simulink model "ball_and_plate_za_nn_2"  (R2018b)
settings: Solver=ode45  StartTime=0.0  StopTime=t_sim  RelTol=1e-3  EnableMultiTasking=on
values from neighbouring files (symbols this model uses):
  A_x = 0.05    [parametri.mat]    (also in proba_nn_simulink.m = 0.1; simulate_NOE_NARX_performance.mat = 0.1; simuliraj_kruznicu.m = radijus; test_nn_.m = 0.1)
  a_x = 0.388    [parametri.mat]    (also in simulate_NOE_NARX_performance.mat)
  A_y = 0.05    [parametri.mat]    (also in proba_nn_simulink.m = 0.1; simulate_NOE_NARX_performance.mat = 0.1; simuliraj_kruznicu.m = radijus; test_nn_.m = 0.1)
  a_y = 0.473    [parametri.mat]    (also in simulate_NOE_NARX_performance.mat)
  Ak_x = 0.1    [parametri.mat]    (also in simulate_NOE_NARX_performance.mat; simuliraj_kvadrat.m = stranica)
  Ak_y = 0.1    [parametri.mat]    (also in simulate_NOE_NARX_performance.mat; simuliraj_kvadrat.m = stranica)
  d = 2    [parametri.mat]    (also in simulate_NOE_NARX_performance.mat)
  Fc = 9.9675e-08    [parametri.mat]    (also in simulate_NOE_NARX_performance.mat)
  freq_x = 0.628318530718    [parametri.mat]    (also in simulate_NOE_NARX_performance.mat)
  freq_y = 0.628318530718    [parametri.mat]    (also in simulate_NOE_NARX_performance.mat)
  Fs = 1.9935e-07    [parametri.mat]    (also in simulate_NOE_NARX_performance.mat)
  g = 9.81    [parametri.mat]    (also in simulate_NOE_NARX_performance.mat)
  Jl = 7.48815837481e-05    [parametri.mat]    (also in simulate_NOE_NARX_performance.mat)
  konstanta = 0.1    [parametri.mat]    (also in simulate_NOE_NARX_performance.mat; simuliraj_kvadrat.m = 0.03)
  l = 0.1    [parametri.mat]    (also in simulate_NOE_NARX_performance.mat)
  ml = 0.0786597330257    [parametri.mat]    (also in simulate_NOE_NARX_performance.mat)
  odabir = 3    [proba_nn_simulink.m]    (also in simulate_NOE_NARX_performance.mat; simuliraj_kruznicu.m; simuliraj_kvadrat.m = 2; simuliraj_referenca.m = 1)
  period_x = 16    [parametri.mat]    (also in simulate_NOE_NARX_performance.mat)
  period_y = 16    [parametri.mat]    (also in simulate_NOE_NARX_performance.mat)
  phase_x = 1.57079632679    [parametri.mat]    (also in simulate_NOE_NARX_performance.mat)
  phase_y = 0    [parametri.mat]    (also in simulate_NOE_NARX_performance.mat)
  phasedelay_x = 0    [parametri.mat]    (also in simulate_NOE_NARX_performance.mat)
  phasedelay_y = 4    [parametri.mat]    (also in simulate_NOE_NARX_performance.mat)
  pw_x = 50    [parametri.mat]    (also in simulate_NOE_NARX_performance.mat)
  pw_y = 50    [parametri.mat]    (also in simulate_NOE_NARX_performance.mat)
  R = 0.0397    [parametri.mat]    (also in simulate_NOE_NARX_performance.mat)
  r = 0.02    [parametri.mat]    (also in simulate_NOE_NARX_performance.mat)
  t_step = 5    [parametri.mat]    (also in simulate_NOE_NARX_performance.mat)
  Td = 0.1    [parametri.mat]    (also in simulate_NOE_NARX_performance.mat)
  vs = 0.05    [parametri.mat]    (also in simulate_NOE_NARX_performance.mat)
  x0 = 0.15    [parametri.mat]    (also in proba_nn_simulink.m = a_x/2.0; simulate_NOE_NARX_performance.mat = 0.194; simuliraj_kruznicu.m = a_x/2.0; test_nn_.m = a_x/2.0)
  x0_loptica = 0.1    [proba_nn_simulink.m]    (also in simulate_NOE_NARX_performance.mat; simuliraj_kruznicu.m = x0_poc; simuliraj_kvadrat.m = x0_poc; simuliraj_referenca.m = x0_poc)
  x_step = 0.05    [parametri.mat]    (also in simulate_NOE_NARX_performance.mat; simuliraj_referenca.m = x_ref_value)
  y0 = 0.15    [parametri.mat]    (also in proba_nn_simulink.m = a_y/2.0; simulate_NOE_NARX_performance.mat = 0.2365; simuliraj_kruznicu.m = a_y/2.0; test_nn_.m = a_y/2.0)
  y0_loptica = 0.1    [proba_nn_simulink.m]    (also in simulate_NOE_NARX_performance.mat; simuliraj_kruznicu.m = y0_poc; simuliraj_kvadrat.m = y0_poc; simuliraj_referenca.m = y0_poc)
  y_step = 0.05    [parametri.mat]    (also in simulate_NOE_NARX_performance.mat; simuliraj_referenca.m = y_ref_value)
libraries: neural x118, simulink x6, fuzblock x2
(part 3 of 5)

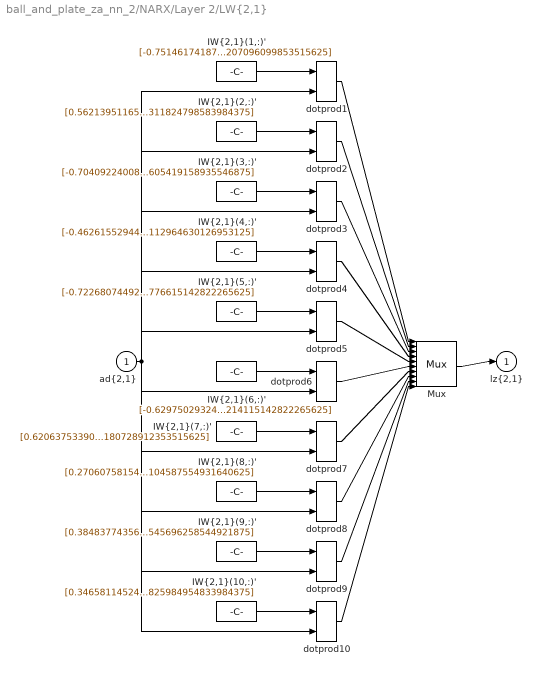
== system ball_and_plate_za_nn_2/NARX/Layer 2/LW{2,1} ==
  "ad{2,1}" : Inport  PortDimensions=10  SampleTime=0.001
      mask Display: e = 0.06;c1 = [120 230 180]/255;c2 = ([120 230 180]+0)/(256+128);c3 = ([120 230 180]+128)/(256+128);patch([0 1 1 0],[0 0 1 1],c1);patch([0 1 1 1-e 1-e 0+e],[0 0 1 1-e 0+e 0+e],c2);patch([0 0 1 1-e 0+e 0+e],[0 1 1 1-e 1-e 0+e],c3);plot([0 1 1 0 0],[0 0 1 1 0]);
  "IW{2,1}(1,:)'" : Constant  Value=[-0.751461741877256894639458550955168902873992919921875;0.01402301635471886638584226858483816613443195819854736328125;0.326442792203841147813392353782546706497669219970703125;0.90660022935466921811809015707694925367832183837890625;-0.407952329174343153450621457523084245622158050537109375;0.609601578751406858458494752994738519191741943359375;-0.255621626399888779435087826641392894089221954345703125;0.10066722871003118411348253857795498333871364593505859375;0.64998266078069499851466161999269388616085052490234375;0.0938512522285636363594818476485670544207096099853515625]
      mask Display: e = 0.06;c1 = [120 150 230]/255;c2 = ([120 150 230]+0)/383;c3 = ([120 150 230]+128)/383;patch([0 1 1 0],[0 0 1 1],c1);patch([0 1 1 1-e 1-e 0+e],[0 0 1 1-e 0+e 0+e],c2);patch([0 0 1 1-e 0+e 0+e],[0 1 1 1-e 1-e 0+e],c3);plot([0 1 1 0 0],[0 0 1 1 0]);disp('weights');
  "IW{2,1}(10,:)'" : Constant  Value=[0.346581145248940847292118405675864778459072113037109375;-0.101987596917314904398921271422295831143856048583984375;-0.199988337664544435501312591441092081367969512939453125;-0.0897556143633064795750442499411292374134063720703125;-0.194407172548844597859130090000689961016178131103515625;-0.8538132542041305672597673037671484053134918212890625;-0.57795138239333410101750132525921799242496490478515625;-0.75194724899415821273152005232986994087696075439453125;-0.5683703056683737653287380453548394143581390380859375;-0.86428952174772832872662320369272492825984954833984375]
      mask Display: e = 0.06;c1 = [120 150 230]/255;c2 = ([120 150 230]+0)/383;c3 = ([120 150 230]+128)/383;patch([0 1 1 0],[0 0 1 1],c1);patch([0 1 1 1-e 1-e 0+e],[0 0 1 1-e 0+e 0+e],c2);patch([0 0 1 1-e 0+e 0+e],[0 1 1 1-e 1-e 0+e],c3);plot([0 1 1 0 0],[0 0 1 1 0]);disp('weights');
  "IW{2,1}(2,:)'" : Constant  Value=[0.56213951165120590314216997285257093608379364013671875;-0.40896438246015787143505804124288260936737060546875;-0.273757397181592476709255379319074563682079315185546875;-0.3103497860711339484396376064978539943695068359375;0.280879223850993786637531002270407043397426605224609375;0.89661471211202348197133460416807793080806732177734375;-0.340117465515137384901578343487926758825778961181640625;-0.249746831523702639277217940616537816822528839111328125;0.572224831191468386037968230084516108036041259765625;0.8546385328160768235505884149461053311824798583984375]
      mask Display: e = 0.06;c1 = [120 150 230]/255;c2 = ([120 150 230]+0)/383;c3 = ([120 150 230]+128)/383;patch([0 1 1 0],[0 0 1 1],c1);patch([0 1 1 1-e 1-e 0+e],[0 0 1 1-e 0+e 0+e],c2);patch([0 0 1 1-e 0+e 0+e],[0 1 1 1-e 1-e 0+e],c3);plot([0 1 1 0 0],[0 0 1 1 0]);disp('weights');
  "IW{2,1}(3,:)'" : Constant  Value=[-0.70409224008847426379276157604181207716464996337890625;0.437857221912158312004947902096319012343883514404296875;0.387908650182214154167326114475145004689693450927734375;-0.313310564539420910445954859824269078671932220458984375;0.5966351041570219226883864394039846956729888916015625;0.25544146338399542628394556231796741485595703125;0.1801270507966407918853946057424764148890972137451171875;-0.1924515838328022809822215322128613479435443878173828125;1.0313756586178184360136356190196238458156585693359375;-0.2004747683477036968024975749358418397605419158935546875]
      mask Display: e = 0.06;c1 = [120 150 230]/255;c2 = ([120 150 230]+0)/383;c3 = ([120 150 230]+128)/383;patch([0 1 1 0],[0 0 1 1],c1);patch([0 1 1 1-e 1-e 0+e],[0 0 1 1-e 0+e 0+e],c2);patch([0 0 1 1-e 0+e 0+e],[0 1 1 1-e 1-e 0+e],c3);plot([0 1 1 0 0],[0 0 1 1 0]);disp('weights');
  "IW{2,1}(4,:)'" : Constant  Value=[-0.46261552944577744028720189817249774932861328125;-0.6083303245955329341398964970721863210201263427734375;0.381563465677544011445121441283845342695713043212890625;0.80056607469864016213279001021874137222766876220703125;0.114817651105901308294932050557690672576427459716796875;-0.31942984216014080889323167866677977144718170166015625;-0.3081261823478540495813149391324259340763092041015625;-0.806724202034220905233041776227764785289764404296875;-0.707544236757142730454006596119143068790435791015625;0.353957390817320860509909152824548073112964630126953125]
      mask Display: e = 0.06;c1 = [120 150 230]/255;c2 = ([120 150 230]+0)/383;c3 = ([120 150 230]+128)/383;patch([0 1 1 0],[0 0 1 1],c1);patch([0 1 1 1-e 1-e 0+e],[0 0 1 1-e 0+e 0+e],c2);patch([0 0 1 1-e 0+e 0+e],[0 1 1 1-e 1-e 0+e],c3);plot([0 1 1 0 0],[0 0 1 1 0]);disp('weights');
  "IW{2,1}(5,:)'" : Constant  Value=[-0.72268074492281775267343846280709840357303619384765625;-0.8099425973058613781319081681431271135807037353515625;-0.48012472297759967165831085367244668304920196533203125;-0.374216308436248923374733976743300445377826690673828125;0.32503796485929414838977891122340224683284759521484375;0.6499760510715775208012701114057563245296478271484375;0.1020332046731853570253889529340085573494434356689453125;-0.51431091597126921133309451761306263506412506103515625;0.2133497896093230483671732145012356340885162353515625;-0.191885414877650595233404828832135535776615142822265625]
      mask Display: e = 0.06;c1 = [120 150 230]/255;c2 = ([120 150 230]+0)/383;c3 = ([120 150 230]+128)/383;patch([0 1 1 0],[0 0 1 1],c1);patch([0 1 1 1-e 1-e 0+e],[0 0 1 1-e 0+e 0+e],c2);patch([0 0 1 1-e 0+e 0+e],[0 1 1 1-e 1-e 0+e],c3);plot([0 1 1 0 0],[0 0 1 1 0]);disp('weights');
  "IW{2,1}(6,:)'" : Constant  Value=[-0.629750293245689096721662281197495758533477783203125;-0.66644903841917801923244724093819968402385711669921875;-0.279327203788677869145118393134907819330692291259765625;-0.440689146090105177133722236249013803899288177490234375;0.309771552515399839489163014150108210742473602294921875;0.460903085493117148363495516605325974524021148681640625;-0.22998472818172943643588723716675303876399993896484375;0.07709746790716941189369748599347076378762722015380859375;-0.1743857796929972614474735337353195063769817352294921875;-0.79638649306433484387213184163556434214115142822265625]
      mask Display: e = 0.06;c1 = [120 150 230]/255;c2 = ([120 150 230]+0)/383;c3 = ([120 150 230]+128)/383;patch([0 1 1 0],[0 0 1 1],c1);patch([0 1 1 1-e 1-e 0+e],[0 0 1 1-e 0+e 0+e],c2);patch([0 0 1 1-e 0+e 0+e],[0 1 1 1-e 1-e 0+e],c3);plot([0 1 1 0 0],[0 0 1 1 0]);disp('weights');
  "IW{2,1}(7,:)'" : Constant  Value=[0.620637533906118310511601521284319460391998291015625;0.83539867376766940854082577061490155756473541259765625;0.27920936398507711917460483164177276194095611572265625;0.7752021630701910748229011005605570971965789794921875;-0.52686260303715248820566330323345027863979339599609375;-0.072403514346486785857592849424690939486026763916015625;-0.05991633433839561873046619666638434864580631256103515625;0.5902810493804420133301391615532338619232177734375;-0.57031874551041517040772532709524966776371002197265625;-0.297717100692596103872489265995682217180728912353515625]
      mask Display: e = 0.06;c1 = [120 150 230]/255;c2 = ([120 150 230]+0)/383;c3 = ([120 150 230]+128)/383;patch([0 1 1 0],[0 0 1 1],c1);patch([0 1 1 1-e 1-e 0+e],[0 0 1 1-e 0+e 0+e],c2);patch([0 0 1 1-e 0+e 0+e],[0 1 1 1-e 1-e 0+e],c3);plot([0 1 1 0 0],[0 0 1 1 0]);disp('weights');
  "IW{2,1}(8,:)'" : Constant  Value=[0.27060758154395336827491291842306964099407196044921875;0.608715135034168408623145296587608754634857177734375;0.55085779675167356739251545150182209908962249755859375;-0.51104733314616945794028879390680231153964996337890625;0.07656481679459646583207899084300152026116847991943359375;0.55887912740008005574310345764388330280780792236328125;-0.37549430899164482067220660610473714768886566162109375;-0.7917369512748544391200766767724417150020599365234375;0.08728549133302436480175146016335929743945598602294921875;0.5207839210335978297194969854899682104587554931640625]
      mask Display: e = 0.06;c1 = [120 150 230]/255;c2 = ([120 150 230]+0)/383;c3 = ([120 150 230]+128)/383;patch([0 1 1 0],[0 0 1 1],c1);patch([0 1 1 1-e 1-e 0+e],[0 0 1 1-e 0+e 0+e],c2);patch([0 0 1 1-e 0+e 0+e],[0 1 1 1-e 1-e 0+e],c3);plot([0 1 1 0 0],[0 0 1 1 0]);disp('weights');
  "IW{2,1}(9,:)'" : Constant  Value=[0.384837743561070311226757212352822534739971160888671875;-0.651296741851778104859249651781283318996429443359375;0.2163767641188421020359555768663994967937469482421875;-0.455812576127146484861185626868973486125469207763671875;-0.91015595086147105252649680551257915794849395751953125;-0.79631028649259560925344203496933914721012115478515625;-0.273943343590692334199587776311091147363185882568359375;0.69205197005795648923509588712477125227451324462890625;0.1748269653888369357108700796743505634367465972900390625;-0.2123389122259488892563439321747864596545696258544921875]
      mask Display: e = 0.06;c1 = [120 150 230]/255;c2 = ([120 150 230]+0)/383;c3 = ([120 150 230]+128)/383;patch([0 1 1 0],[0 0 1 1],c1);patch([0 1 1 1-e 1-e 0+e],[0 0 1 1-e 0+e 0+e],c2);patch([0 0 1 1-e 0+e 0+e],[0 1 1 1-e 1-e 0+e],c3);plot([0 1 1 0 0],[0 0 1 1 0]);disp('weights');
  Mux : Mux  Inputs=10
      mask Display: e = 0.06;c1 = [120 150 230]/255;c2 = ([120 150 230]+0)/383;c3 = ([120 150 230]+128)/383;patch([0 1 1 0],[0 0 1 1],c1);patch([0 1 1 1-e 1-e 0+e],[0 0 1 1-e 0+e 0+e],c2);patch([0 0 1 1-e 0+e 0+e],[0 1 1 1-e 1-e 0+e],c3);plot([0 1 1 0 0],[0 0 1 1 0]);disp('Mux');
  dotprod{1..10} (10 alike) : neural/Weight Functions/dotprod
  "lz{2,1}" : Outport
      mask Display: e = 0.06;c1 = [120 230 180]/255;c2 = ([120 230 180]+0)/(256+128);c3 = ([120 230 180]+128)/(256+128);patch([0 1 1 0],[0 0 1 1],c1);patch([0 1 1 1-e 1-e 0+e],[0 0 1 1-e 0+e 0+e],c2);patch([0 0 1 1-e 0+e 0+e],[0 1 1 1-e 1-e 0+e],c3);plot([0 1 1 0 0],[0 0 1 1 0]);
  wires:
  "IW{2,1}(1,:)'"/1 -> dotprod1/1
  "ad{2,1}"/1 -> dotprod1/2, dotprod2/2, dotprod3/2, dotprod4/2, dotprod5/2, dotprod6/2, dotprod7/2, dotprod8/2, dotprod9/2, dotprod10/2
  dotprod1/1 -> Mux/1
  "IW{2,1}(2,:)'"/1 -> dotprod2/1
  dotprod2/1 -> Mux/2
  "IW{2,1}(3,:)'"/1 -> dotprod3/1
  dotprod3/1 -> Mux/3
  "IW{2,1}(4,:)'"/1 -> dotprod4/1
  dotprod4/1 -> Mux/4
  "IW{2,1}(5,:)'"/1 -> dotprod5/1
  dotprod5/1 -> Mux/5
  "IW{2,1}(6,:)'"/1 -> dotprod6/1
  dotprod6/1 -> Mux/6
  "IW{2,1}(7,:)'"/1 -> dotprod7/1
  dotprod7/1 -> Mux/7
  "IW{2,1}(8,:)'"/1 -> dotprod8/1
  dotprod8/1 -> Mux/8
  "IW{2,1}(9,:)'"/1 -> dotprod9/1
  dotprod9/1 -> Mux/9
  "IW{2,1}(10,:)'"/1 -> dotprod10/1
  dotprod10/1 -> Mux/10
  Mux/1 -> "lz{2,1}"/1

== system ball_and_plate_za_nn_2/NARX/Layer 3/Delays 1 ==
  "p{3}" : Inport  PortDimensions=10  SampleTime=0.001
      mask Display: e = 0.06;c1 = [120 230 180]/255;c2 = ([120 230 180]+0)/(256+128);c3 = ([120 230 180]+128)/(256+128);patch([0 1 1 0],[0 0 1 1],c1);patch([0 1 1 1-e 1-e 0+e],[0 0 1 1-e 0+e 0+e],c2);patch([0 0 1 1-e 0+e 0+e],[0 1 1 1-e 1-e 0+e],c3);plot([0 1 1 0 0],[0 0 1 1 0]);
  mux : Mux  Inputs=1
      mask Display: e = 0.06;c1 = [120 150 230]/255;c2 = ([120 150 230]+0)/383;c3 = ([120 150 230]+128)/383;patch([0 1 1 0],[0 0 1 1],c1);patch([0 1 1 1-e 1-e 0+e],[0 0 1 1-e 0+e 0+e],c2);patch([0 0 1 1-e 0+e 0+e],[0 1 1 1-e 1-e 0+e],c3);plot([0 1 1 0 0],[0 0 1 1 0]);disp('Mux')
  "pd{3,2}" : Outport
      mask Display: e = 0.06;c1 = [120 230 180]/255;c2 = ([120 230 180]+0)/(256+128);c3 = ([120 230 180]+128)/(256+128);patch([0 1 1 0],[0 0 1 1],c1);patch([0 1 1 1-e 1-e 0+e],[0 0 1 1-e 0+e 0+e],c2);patch([0 0 1 1-e 0+e 0+e],[0 1 1 1-e 1-e 0+e],c3);plot([0 1 1 0 0],[0 0 1 1 0]);
  wires:
  "p{3}"/1 -> mux/1
  mux/1 -> "pd{3,2}"/1

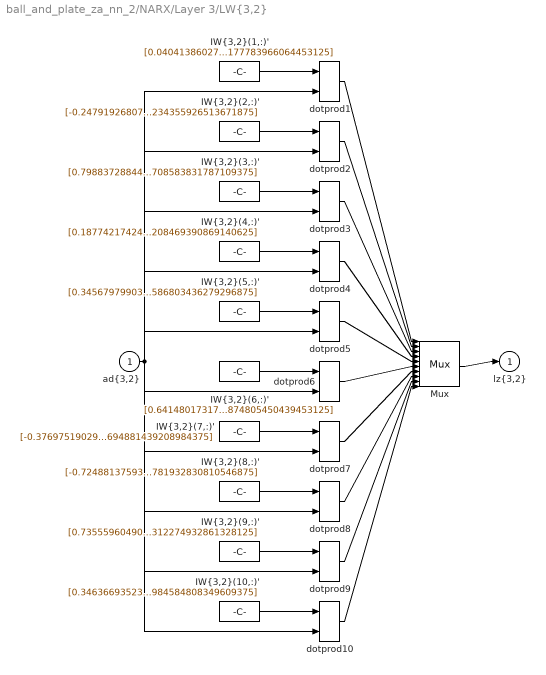
== system ball_and_plate_za_nn_2/NARX/Layer 3/LW{3,2} ==
  "ad{3,2}" : Inport  PortDimensions=10  SampleTime=0.001
      mask Display: e = 0.06;c1 = [120 230 180]/255;c2 = ([120 230 180]+0)/(256+128);c3 = ([120 230 180]+128)/(256+128);patch([0 1 1 0],[0 0 1 1],c1);patch([0 1 1 1-e 1-e 0+e],[0 0 1 1-e 0+e 0+e],c2);patch([0 0 1 1-e 0+e 0+e],[0 1 1 1-e 1-e 0+e],c3);plot([0 1 1 0 0],[0 0 1 1 0]);
  "IW{3,2}(1,:)'" : Constant  Value=[0.040413860274551162421463601504001417197287082672119140625;-0.922390700485416825671336482628248631954193115234375;-0.2847704915836410943796863648458383977413177490234375;-0.119375039110782898976736987606273032724857330322265625;-0.341439083972712775771896076548728160560131072998046875;-0.50733485064919781049042057929909788072109222412109375;0.8200616320720737206784178852103650569915771484375;-0.503983609435054713543422622024081647396087646484375;-0.57818123350426275930402653102646581828594207763671875;-0.64161556160537447368596986052580177783966064453125]
      mask Display: e = 0.06;c1 = [120 150 230]/255;c2 = ([120 150 230]+0)/383;c3 = ([120 150 230]+128)/383;patch([0 1 1 0],[0 0 1 1],c1);patch([0 1 1 1-e 1-e 0+e],[0 0 1 1-e 0+e 0+e],c2);patch([0 0 1 1-e 0+e 0+e],[0 1 1 1-e 1-e 0+e],c3);plot([0 1 1 0 0],[0 0 1 1 0]);disp('weights');
  "IW{3,2}(10,:)'" : Constant  Value=[0.346366935233423045570333442810806445777416229248046875;0.57982113783220901037651628939784131944179534912109375;0.57340249697952316854099308329750783741474151611328125;-0.63663622611961334651908828163868747651576995849609375;0.493057047298153694470101982005871832370758056640625;-0.61295474090280033241384671782725490629673004150390625;-0.307687812221070278173584711112198419868946075439453125;0.889968060640594416099702357314527034759521484375;0.218127843394698761603223147176322527229785919189453125;0.594582300739323610372366601950488984584808349609375]
      mask Display: e = 0.06;c1 = [120 150 230]/255;c2 = ([120 150 230]+0)/383;c3 = ([120 150 230]+128)/383;patch([0 1 1 0],[0 0 1 1],c1);patch([0 1 1 1-e 1-e 0+e],[0 0 1 1-e 0+e 0+e],c2);patch([0 0 1 1-e 0+e 0+e],[0 1 1 1-e 1-e 0+e],c3);plot([0 1 1 0 0],[0 0 1 1 0]);disp('weights');
  "IW{3,2}(2,:)'" : Constant  Value=[-0.247919268078307719616049098476651124656200408935546875;0.94436124925423892140230464065098203718662261962890625;0.9270543276709377611410900499322451651096343994140625;-0.392239860060123957108402237281552515923976898193359375;-0.28425051274919932442486469881259836256504058837890625;0.482043595032938976263636732255690731108188629150390625;0.055639342668838687178123336707358248531818389892578125;-0.596649201567405196300342140602879226207733154296875;0.30360672151137746421767360516241751611232757568359375;0.55585618915527390537789642621646635234355926513671875]
      mask Display: e = 0.06;c1 = [120 150 230]/255;c2 = ([120 150 230]+0)/383;c3 = ([120 150 230]+128)/383;patch([0 1 1 0],[0 0 1 1],c1);patch([0 1 1 1-e 1-e 0+e],[0 0 1 1-e 0+e 0+e],c2);patch([0 0 1 1-e 0+e 0+e],[0 1 1 1-e 1-e 0+e],c3);plot([0 1 1 0 0],[0 0 1 1 0]);disp('weights');
  "IW{3,2}(3,:)'" : Constant  Value=[0.7988372884423233788453444503829814493656158447265625;0.10264407291714987280339954622832010500133037567138671875;-0.30225989466886293843828070748713798820972442626953125;1.28639752379728378173240344040095806121826171875;0.555473538436132230344810523092746734619140625;0.258883734010433685934771119718789122998714447021484375;-0.6018171316378688739945346242166124284267425537109375;0.155025731162292956799575449622352607548236846923828125;0.1034283261229422823390677876886911690235137939453125;0.0768932827783828931611509460708475671708583831787109375]
      mask Display: e = 0.06;c1 = [120 150 230]/255;c2 = ([120 150 230]+0)/383;c3 = ([120 150 230]+128)/383;patch([0 1 1 0],[0 0 1 1],c1);patch([0 1 1 1-e 1-e 0+e],[0 0 1 1-e 0+e 0+e],c2);patch([0 0 1 1-e 0+e 0+e],[0 1 1 1-e 1-e 0+e],c3);plot([0 1 1 0 0],[0 0 1 1 0]);disp('weights');
  "IW{3,2}(4,:)'" : Constant  Value=[0.1877421742496100109942602784940390847623348236083984375;0.073772548326666242957116992329247295856475830078125;0.98389896042601099335200842688209377229213714599609375;0.1587567177918024763361160012209438718855381011962890625;-0.68414865746699071724634677593712694942951202392578125;0.90332478490211898236594834088464267551898956298828125;0.0626931921731869457037333859261707402765750885009765625;-0.047387286905901500333460063529855688102543354034423828125;-0.7018867120396026226814001347520388662815093994140625;-0.409896420558823637581014054376282729208469390869140625]
      mask Display: e = 0.06;c1 = [120 150 230]/255;c2 = ([120 150 230]+0)/383;c3 = ([120 150 230]+128)/383;patch([0 1 1 0],[0 0 1 1],c1);patch([0 1 1 1-e 1-e 0+e],[0 0 1 1-e 0+e 0+e],c2);patch([0 0 1 1-e 0+e 0+e],[0 1 1 1-e 1-e 0+e],c3);plot([0 1 1 0 0],[0 0 1 1 0]);disp('weights');
  "IW{3,2}(5,:)'" : Constant  Value=[0.34567979903814627373748180616530589759349822998046875;0.1689745227071446087574457806113059632480144500732421875;-0.65511477638029180781131799449212849140167236328125;-0.06799106151517965435093771020547137595713138580322265625;0.94811307052564597341870467062108218669891357421875;0.17434245159570094241274773594341240823268890380859375;0.399634533379687739707009086487232707440853118896484375;0.230065935698102574935575148629141040146350860595703125;-0.93213216556273181812031225490500219166278839111328125;0.8302746033940511249937799220788292586803436279296875]
      mask Display: e = 0.06;c1 = [120 150 230]/255;c2 = ([120 150 230]+0)/383;c3 = ([120 150 230]+128)/383;patch([0 1 1 0],[0 0 1 1],c1);patch([0 1 1 1-e 1-e 0+e],[0 0 1 1-e 0+e 0+e],c2);patch([0 0 1 1-e 0+e 0+e],[0 1 1 1-e 1-e 0+e],c3);plot([0 1 1 0 0],[0 0 1 1 0]);disp('weights');
  "IW{3,2}(6,:)'" : Constant  Value=[0.64148017317841821149926317957579158246517181396484375;0.371266902779530116873729639337398111820220947265625;-0.54654195876076572258028818396269343793392181396484375;-0.6314329269674636702092129780794493854045867919921875;-0.69913434240755389925681129170698113739490509033203125;0.70557959923069846208676381138502620160579681396484375;0.007333167928958259952632037226294414722360670566558837890625;-0.5018673974887419841905966677586548030376434326171875;0.5595800924386253871745111609925515949726104736328125;0.463373418118516344765822623230633325874805450439453125]
      mask Display: e = 0.06;c1 = [120 150 230]/255;c2 = ([120 150 230]+0)/383;c3 = ([120 150 230]+128)/383;patch([0 1 1 0],[0 0 1 1],c1);patch([0 1 1 1-e 1-e 0+e],[0 0 1 1-e 0+e 0+e],c2);patch([0 0 1 1-e 0+e 0+e],[0 1 1 1-e 1-e 0+e],c3);plot([0 1 1 0 0],[0 0 1 1 0]);disp('weights');
  "IW{3,2}(7,:)'" : Constant  Value=[-0.3769751902976870017170085702673532068729400634765625;0.74558407385953240353870796752744354307651519775390625;0.82763245776990423951957609460805542767047882080078125;-0.351946351905890908451368659370928071439266204833984375;-0.054512753614597987683598745434210286475718021392822265625;0.1042060761942014968095548965720809064805507659912109375;-0.3220293929206798910769293797784484922885894775390625;0.74298526277768084380426216739579103887081146240234375;0.478710071650852331259784477879293262958526611328125;0.65508440118354316350490762488334439694881439208984375]
      mask Display: e = 0.06;c1 = [120 150 230]/255;c2 = ([120 150 230]+0)/383;c3 = ([120 150 230]+128)/383;patch([0 1 1 0],[0 0 1 1],c1);patch([0 1 1 1-e 1-e 0+e],[0 0 1 1-e 0+e 0+e],c2);patch([0 0 1 1-e 0+e 0+e],[0 1 1 1-e 1-e 0+e],c3);plot([0 1 1 0 0],[0 0 1 1 0]);disp('weights');
  "IW{3,2}(8,:)'" : Constant  Value=[-0.724881375936054173081402041134424507617950439453125;-0.224228758994157562067783828751998953521251678466796875;-0.878991633763001711798779069795273244380950927734375;-0.34410970441512434003783482694416306912899017333984375;-0.796031048304059130060750248958356678485870361328125;-0.28685401288189849022813859846792183816432952880859375;0.597673707986199342911959320190362632274627685546875;0.204473374062566104480964668255182914435863494873046875;-0.12496619004476315628604510266086435876786708831787109375;-0.72977447209500478919608212891034781932830810546875]
      mask Display: e = 0.06;c1 = [120 150 230]/255;c2 = ([120 150 230]+0)/383;c3 = ([120 150 230]+128)/383;patch([0 1 1 0],[0 0 1 1],c1);patch([0 1 1 1-e 1-e 0+e],[0 0 1 1-e 0+e 0+e],c2);patch([0 0 1 1-e 0+e 0+e],[0 1 1 1-e 1-e 0+e],c3);plot([0 1 1 0 0],[0 0 1 1 0]);disp('weights');
  "IW{3,2}(9,:)'" : Constant  Value=[0.7355596049033739092237738077528774738311767578125;-0.61561420101332864351917351086740382015705108642578125;0.63945812650363631490790794487111270427703857421875;0.39810918430234931708611156864208169281482696533203125;0.45761704785750267898691845402936451137065887451171875;-0.01410886982849469777068218689919376629404723644256591796875;0.464929409371541313422682151212939061224460601806640625;-0.065512359979736423110097121025319211184978485107421875;-0.63074968859026470102691064312239177525043487548828125;-0.5151336803297141830881855639745481312274932861328125]
      mask Display: e = 0.06;c1 = [120 150 230]/255;c2 = ([120 150 230]+0)/383;c3 = ([120 150 230]+128)/383;patch([0 1 1 0],[0 0 1 1],c1);patch([0 1 1 1-e 1-e 0+e],[0 0 1 1-e 0+e 0+e],c2);patch([0 0 1 1-e 0+e 0+e],[0 1 1 1-e 1-e 0+e],c3);plot([0 1 1 0 0],[0 0 1 1 0]);disp('weights');
  Mux : Mux  Inputs=10
      mask Display: e = 0.06;c1 = [120 150 230]/255;c2 = ([120 150 230]+0)/383;c3 = ([120 150 230]+128)/383;patch([0 1 1 0],[0 0 1 1],c1);patch([0 1 1 1-e 1-e 0+e],[0 0 1 1-e 0+e 0+e],c2);patch([0 0 1 1-e 0+e 0+e],[0 1 1 1-e 1-e 0+e],c3);plot([0 1 1 0 0],[0 0 1 1 0]);disp('Mux');
  dotprod{1..10} (10 alike) : neural/Weight Functions/dotprod
  "lz{3,2}" : Outport
      mask Display: e = 0.06;c1 = [120 230 180]/255;c2 = ([120 230 180]+0)/(256+128);c3 = ([120 230 180]+128)/(256+128);patch([0 1 1 0],[0 0 1 1],c1);patch([0 1 1 1-e 1-e 0+e],[0 0 1 1-e 0+e 0+e],c2);patch([0 0 1 1-e 0+e 0+e],[0 1 1 1-e 1-e 0+e],c3);plot([0 1 1 0 0],[0 0 1 1 0]);
  wires:
  "IW{3,2}(1,:)'"/1 -> dotprod1/1
  "ad{3,2}"/1 -> dotprod1/2, dotprod2/2, dotprod3/2, dotprod4/2, dotprod5/2, dotprod6/2, dotprod7/2, dotprod8/2, dotprod9/2, dotprod10/2
  dotprod1/1 -> Mux/1
  "IW{3,2}(2,:)'"/1 -> dotprod2/1
  dotprod2/1 -> Mux/2
  "IW{3,2}(3,:)'"/1 -> dotprod3/1
  dotprod3/1 -> Mux/3
  "IW{3,2}(4,:)'"/1 -> dotprod4/1
  dotprod4/1 -> Mux/4
  "IW{3,2}(5,:)'"/1 -> dotprod5/1
  dotprod5/1 -> Mux/5
  "IW{3,2}(6,:)'"/1 -> dotprod6/1
  dotprod6/1 -> Mux/6
  "IW{3,2}(7,:)'"/1 -> dotprod7/1
  dotprod7/1 -> Mux/7
  "IW{3,2}(8,:)'"/1 -> dotprod8/1
  dotprod8/1 -> Mux/8
  "IW{3,2}(9,:)'"/1 -> dotprod9/1
  dotprod9/1 -> Mux/9
  "IW{3,2}(10,:)'"/1 -> dotprod10/1
  dotprod10/1 -> Mux/10
  Mux/1 -> "lz{3,2}"/1

== system ball_and_plate_za_nn_2/NARX/Layer 4/Delays 1 ==
  "p{4}" : Inport  PortDimensions=10  SampleTime=0.001
      mask Display: e = 0.06;c1 = [120 230 180]/255;c2 = ([120 230 180]+0)/(256+128);c3 = ([120 230 180]+128)/(256+128);patch([0 1 1 0],[0 0 1 1],c1);patch([0 1 1 1-e 1-e 0+e],[0 0 1 1-e 0+e 0+e],c2);patch([0 0 1 1-e 0+e 0+e],[0 1 1 1-e 1-e 0+e],c3);plot([0 1 1 0 0],[0 0 1 1 0]);
  mux : Mux  Inputs=1
      mask Display: e = 0.06;c1 = [120 150 230]/255;c2 = ([120 150 230]+0)/383;c3 = ([120 150 230]+128)/383;patch([0 1 1 0],[0 0 1 1],c1);patch([0 1 1 1-e 1-e 0+e],[0 0 1 1-e 0+e 0+e],c2);patch([0 0 1 1-e 0+e 0+e],[0 1 1 1-e 1-e 0+e],c3);plot([0 1 1 0 0],[0 0 1 1 0]);disp('Mux')
  "pd{4,3}" : Outport
      mask Display: e = 0.06;c1 = [120 230 180]/255;c2 = ([120 230 180]+0)/(256+128);c3 = ([120 230 180]+128)/(256+128);patch([0 1 1 0],[0 0 1 1],c1);patch([0 1 1 1-e 1-e 0+e],[0 0 1 1-e 0+e 0+e],c2);patch([0 0 1 1-e 0+e 0+e],[0 1 1 1-e 1-e 0+e],c3);plot([0 1 1 0 0],[0 0 1 1 0]);
  wires:
  "p{4}"/1 -> mux/1
  mux/1 -> "pd{4,3}"/1

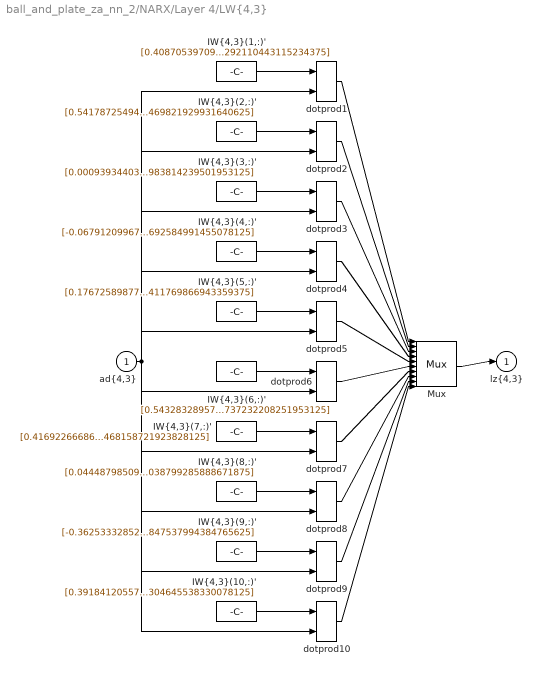
== system ball_and_plate_za_nn_2/NARX/Layer 4/LW{4,3} ==
  "ad{4,3}" : Inport  PortDimensions=10  SampleTime=0.001
      mask Display: e = 0.06;c1 = [120 230 180]/255;c2 = ([120 230 180]+0)/(256+128);c3 = ([120 230 180]+128)/(256+128);patch([0 1 1 0],[0 0 1 1],c1);patch([0 1 1 1-e 1-e 0+e],[0 0 1 1-e 0+e 0+e],c2);patch([0 0 1 1-e 0+e 0+e],[0 1 1 1-e 1-e 0+e],c3);plot([0 1 1 0 0],[0 0 1 1 0]);
  "IW{4,3}(1,:)'" : Constant  Value=[0.40870539709809461381695427917293272912502288818359375;-0.2540888691627125606231629717512987554073333740234375;-0.57666466027429830187855941403540782630443572998046875;-0.80617111640670457983759433773229829967021942138671875;-0.3095025876504846618075816877535544335842132568359375;0.01232055950833396869292801767414857749827206134796142578125;0.91501847459988361332960948857362382113933563232421875;0.046476927022480130080595017716404981911182403564453125;-0.78709696630178560550206157131469808518886566162109375;0.2299334424622970496354668057392700575292110443115234375]
      mask Display: e = 0.06;c1 = [120 150 230]/255;c2 = ([120 150 230]+0)/383;c3 = ([120 150 230]+128)/383;patch([0 1 1 0],[0 0 1 1],c1);patch([0 1 1 1-e 1-e 0+e],[0 0 1 1-e 0+e 0+e],c2);patch([0 0 1 1-e 0+e 0+e],[0 1 1 1-e 1-e 0+e],c3);plot([0 1 1 0 0],[0 0 1 1 0]);disp('weights');
  "IW{4,3}(10,:)'" : Constant  Value=[0.391841205571248296646302833323716185986995697021484375;-0.77287431052964972177932168051484040915966033935546875;-0.2218660454561571515608164872901397757232189178466796875;-0.9501743690746662363011409979662857949733734130859375;-0.1314231945874096141313458474542130716145038604736328125;0.575969759172148432213589330785907804965972900390625;-0.50019731440796999510922660192591138184070587158203125;0.8354966701444543897281391764408908784389495849609375;-0.266684952879488401666918662158423103392124176025390625;0.60316473971497963635357564271544106304645538330078125]
      mask Display: e = 0.06;c1 = [120 150 230]/255;c2 = ([120 150 230]+0)/383;c3 = ([120 150 230]+128)/383;patch([0 1 1 0],[0 0 1 1],c1);patch([0 1 1 1-e 1-e 0+e],[0 0 1 1-e 0+e 0+e],c2);patch([0 0 1 1-e 0+e 0+e],[0 1 1 1-e 1-e 0+e],c3);plot([0 1 1 0 0],[0 0 1 1 0]);disp('weights');
  "IW{4,3}(2,:)'" : Constant  Value=[0.5417872549415123639704461311339400708675384521484375;0.26188639563861493275709335648571141064167022705078125;-1.060594195346266754853559177718125283718109130859375;-0.048002513012465684860696768510024412535130977630615234375;-0.1780902217946197796383245304241427220404148101806640625;0.054981556481401593072799727224264643155038356781005859375;-0.81666236417747395393007536767981946468353271484375;0.38904090476776287399474085759720765054225921630859375;-0.939386293784676862372862160555087029933929443359375;0.24049926258863651984398757122107781469821929931640625]
      mask Display: e = 0.06;c1 = [120 150 230]/255;c2 = ([120 150 230]+0)/383;c3 = ([120 150 230]+128)/383;patch([0 1 1 0],[0 0 1 1],c1);patch([0 1 1 1-e 1-e 0+e],[0 0 1 1-e 0+e 0+e],c2);patch([0 0 1 1-e 0+e 0+e],[0 1 1 1-e 1-e 0+e],c3);plot([0 1 1 0 0],[0 0 1 1 0]);disp('weights');
  "IW{4,3}(3,:)'" : Constant  Value=[0.000939344033684942798789752060883984086103737354278564453125;0.84524127369610091431439968800987116992473602294921875;-0.3941174691466595714217646673205308616161346435546875;1.0034068425839268723365194091456942260265350341796875;0.231753049913562048089943345985375344753265380859375;-0.5192550117031713430293393685133196413516998291015625;-0.208887211309706610773417878590407781302928924560546875;0.28539820305701379954399499183637090027332305908203125;0.77759269305989831000403000871301628649234771728515625;0.381779872290980482052447086971369571983814239501953125]
      mask Display: e = 0.06;c1 = [120 150 230]/255;c2 = ([120 150 230]+0)/383;c3 = ([120 150 230]+128)/383;patch([0 1 1 0],[0 0 1 1],c1);patch([0 1 1 1-e 1-e 0+e],[0 0 1 1-e 0+e 0+e],c2);patch([0 0 1 1-e 0+e 0+e],[0 1 1 1-e 1-e 0+e],c3);plot([0 1 1 0 0],[0 0 1 1 0]);disp('weights');
  "IW{4,3}(4,:)'" : Constant  Value=[-0.06791209967671564540214745875346125103533267974853515625;0.66430400356172680798039209548733197152614593505859375;-0.25316358100225777594260989644681103527545928955078125;-0.351702647292925385524853254537447355687618255615234375;0.87479107515515075466083771971170790493488311767578125;-0.94018974009686306914090891950763761997222900390625;0.795091425512663096952792329830117523670196533203125;0.210380897711272163430606951806112192571163177490234375;-0.5296542738384466542100881270016543567180633544921875;0.2220539022214716162739733817943488247692584991455078125]
      mask Display: e = 0.06;c1 = [120 150 230]/255;c2 = ([120 150 230]+0)/383;c3 = ([120 150 230]+128)/383;patch([0 1 1 0],[0 0 1 1],c1);patch([0 1 1 1-e 1-e 0+e],[0 0 1 1-e 0+e 0+e],c2);patch([0 0 1 1-e 0+e 0+e],[0 1 1 1-e 1-e 0+e],c3);plot([0 1 1 0 0],[0 0 1 1 0]);disp('weights');
  "IW{4,3}(5,:)'" : Constant  Value=[0.1767258987712781170831277677280013449490070343017578125;0.91630858276520676941601095677469857037067413330078125;0.2007543073089513574469577861236757598817348480224609375;0.154980445589328663658079676679335534572601318359375;-0.1683306701251934267560272928676567971706390380859375;-0.84826572881355699617955679059377871453762054443359375;0.293111189214277256809282334870658814907073974609375;-0.20264528265917858274036689181230030953884124755859375;-1.01057004139361961136955869733355939388275146484375;-0.08291356458034003507062692506224266253411769866943359375]
      mask Display: e = 0.06;c1 = [120 150 230]/255;c2 = ([120 150 230]+0)/383;c3 = ([120 150 230]+128)/383;patch([0 1 1 0],[0 0 1 1],c1);patch([0 1 1 1-e 1-e 0+e],[0 0 1 1-e 0+e 0+e],c2);patch([0 0 1 1-e 0+e 0+e],[0 1 1 1-e 1-e 0+e],c3);plot([0 1 1 0 0],[0 0 1 1 0]);disp('weights');
  "IW{4,3}(6,:)'" : Constant  Value=[0.54328328957335891846724962306325323879718780517578125;0.691608251953872876782725143129937350749969482421875;0.6078641552083838828224315875559113919734954833984375;0.25679773545168027570895219469093717634677886962890625;-0.054190034319975328991336738226891611702740192413330078125;0.6238359561945963083218202882562763988971710205078125;0.81508785066547806419379185172147117555141448974609375;-0.453777327654840856308027241539093665778636932373046875;0.56547815556141733939199411906884051859378814697265625;-0.5938651505074663550232116904226131737232208251953125]
      mask Display: e = 0.06;c1 = [120 150 230]/255;c2 = ([120 150 230]+0)/383;c3 = ([120 150 230]+128)/383;patch([0 1 1 0],[0 0 1 1],c1);patch([0 1 1 1-e 1-e 0+e],[0 0 1 1-e 0+e 0+e],c2);patch([0 0 1 1-e 0+e 0+e],[0 1 1 1-e 1-e 0+e],c3);plot([0 1 1 0 0],[0 0 1 1 0]);disp('weights');
  "IW{4,3}(7,:)'" : Constant  Value=[0.416922666869295743818923938306397758424282073974609375;0.79366518187884260715492246163194067776203155517578125;-0.484883128064957535929835330534842796623706817626953125;-0.1164025271941328265601356406477862037718296051025390625;0.6113968684917006068957334719016216695308685302734375;-0.66721431902438299577084990232833661139011383056640625;-0.044172263035992830049192292563020600937306880950927734375;-0.1867029155844549814791122344104223884642124176025390625;-0.88087186787475157956350813037715852260589599609375;0.63456291886210280939195627070148475468158721923828125]
      mask Display: e = 0.06;c1 = [120 150 230]/255;c2 = ([120 150 230]+0)/383;c3 = ([120 150 230]+128)/383;patch([0 1 1 0],[0 0 1 1],c1);patch([0 1 1 1-e 1-e 0+e],[0 0 1 1-e 0+e 0+e],c2);patch([0 0 1 1-e 0+e 0+e],[0 1 1 1-e 1-e 0+e],c3);plot([0 1 1 0 0],[0 0 1 1 0]);disp('weights');
  "IW{4,3}(8,:)'" : Constant  Value=[0.044487985093605221520451920014238567091524600982666015625;-0.8464129571423535391971881836070679128170013427734375;-0.10913072854795903554592229056652286089956760406494140625;-0.1547982046578038894946161008192575536668300628662109375;-0.1417084793712377333019247771517257206141948699951171875;0.5689093401124012405745133946766145527362823486328125;-0.85969885445430749282280658007948659360408782958984375;-0.8234758079399835395406626048497855663299560546875;0.64619184530852680214962902027764357626438140869140625;-0.445754039863237749852231672775815241038799285888671875]
      mask Display: e = 0.06;c1 = [120 150 230]/255;c2 = ([120 150 230]+0)/383;c3 = ([120 150 230]+128)/383;patch([0 1 1 0],[0 0 1 1],c1);patch([0 1 1 1-e 1-e 0+e],[0 0 1 1-e 0+e 0+e],c2);patch([0 0 1 1-e 0+e 0+e],[0 1 1 1-e 1-e 0+e],c3);plot([0 1 1 0 0],[0 0 1 1 0]);disp('weights');
  "IW{4,3}(9,:)'" : Constant  Value=[-0.36253332852955555409835142199881374835968017578125;-0.86417254264218901216310086965677328407764434814453125;0.61938491178412935500574576508370228111743927001953125;0.79094265482623649088367301374091766774654388427734375;0.63959137502408525133290595476864837110042572021484375;0.382269537268440540156433371521416120231151580810546875;0.2201585580218360649329412126462557353079319000244140625;0.1824392069742414579369693683474906720221042633056640625;-0.70387644815780425755491478412295691668987274169921875;0.27393026557719812874580611605779267847537994384765625]
      mask Display: e = 0.06;c1 = [120 150 230]/255;c2 = ([120 150 230]+0)/383;c3 = ([120 150 230]+128)/383;patch([0 1 1 0],[0 0 1 1],c1);patch([0 1 1 1-e 1-e 0+e],[0 0 1 1-e 0+e 0+e],c2);patch([0 0 1 1-e 0+e 0+e],[0 1 1 1-e 1-e 0+e],c3);plot([0 1 1 0 0],[0 0 1 1 0]);disp('weights');
  Mux : Mux  Inputs=10
      mask Display: e = 0.06;c1 = [120 150 230]/255;c2 = ([120 150 230]+0)/383;c3 = ([120 150 230]+128)/383;patch([0 1 1 0],[0 0 1 1],c1);patch([0 1 1 1-e 1-e 0+e],[0 0 1 1-e 0+e 0+e],c2);patch([0 0 1 1-e 0+e 0+e],[0 1 1 1-e 1-e 0+e],c3);plot([0 1 1 0 0],[0 0 1 1 0]);disp('Mux');
  dotprod{1..10} (10 alike) : neural/Weight Functions/dotprod
  "lz{4,3}" : Outport
      mask Display: e = 0.06;c1 = [120 230 180]/255;c2 = ([120 230 180]+0)/(256+128);c3 = ([120 230 180]+128)/(256+128);patch([0 1 1 0],[0 0 1 1],c1);patch([0 1 1 1-e 1-e 0+e],[0 0 1 1-e 0+e 0+e],c2);patch([0 0 1 1-e 0+e 0+e],[0 1 1 1-e 1-e 0+e],c3);plot([0 1 1 0 0],[0 0 1 1 0]);
  wires:
  "IW{4,3}(1,:)'"/1 -> dotprod1/1
  "ad{4,3}"/1 -> dotprod1/2, dotprod2/2, dotprod3/2, dotprod4/2, dotprod5/2, dotprod6/2, dotprod7/2, dotprod8/2, dotprod9/2, dotprod10/2
  dotprod1/1 -> Mux/1
  "IW{4,3}(2,:)'"/1 -> dotprod2/1
  dotprod2/1 -> Mux/2
  "IW{4,3}(3,:)'"/1 -> dotprod3/1
  dotprod3/1 -> Mux/3
  "IW{4,3}(4,:)'"/1 -> dotprod4/1
  dotprod4/1 -> Mux/4
  "IW{4,3}(5,:)'"/1 -> dotprod5/1
  dotprod5/1 -> Mux/5
  "IW{4,3}(6,:)'"/1 -> dotprod6/1
  dotprod6/1 -> Mux/6
  "IW{4,3}(7,:)'"/1 -> dotprod7/1
  dotprod7/1 -> Mux/7
  "IW{4,3}(8,:)'"/1 -> dotprod8/1
  dotprod8/1 -> Mux/8
  "IW{4,3}(9,:)'"/1 -> dotprod9/1
  dotprod9/1 -> Mux/9
  "IW{4,3}(10,:)'"/1 -> dotprod10/1
  dotprod10/1 -> Mux/10
  Mux/1 -> "lz{4,3}"/1

== system ball_and_plate_za_nn_2/NARX/Layer 5/Delays 1 ==
  "p{5}" : Inport  PortDimensions=10  SampleTime=0.001
      mask Display: e = 0.06;c1 = [120 230 180]/255;c2 = ([120 230 180]+0)/(256+128);c3 = ([120 230 180]+128)/(256+128);patch([0 1 1 0],[0 0 1 1],c1);patch([0 1 1 1-e 1-e 0+e],[0 0 1 1-e 0+e 0+e],c2);patch([0 0 1 1-e 0+e 0+e],[0 1 1 1-e 1-e 0+e],c3);plot([0 1 1 0 0],[0 0 1 1 0]);
  mux : Mux  Inputs=1
      mask Display: e = 0.06;c1 = [120 150 230]/255;c2 = ([120 150 230]+0)/383;c3 = ([120 150 230]+128)/383;patch([0 1 1 0],[0 0 1 1],c1);patch([0 1 1 1-e 1-e 0+e],[0 0 1 1-e 0+e 0+e],c2);patch([0 0 1 1-e 0+e 0+e],[0 1 1 1-e 1-e 0+e],c3);plot([0 1 1 0 0],[0 0 1 1 0]);disp('Mux')
  "pd{5,4}" : Outport
      mask Display: e = 0.06;c1 = [120 230 180]/255;c2 = ([120 230 180]+0)/(256+128);c3 = ([120 230 180]+128)/(256+128);patch([0 1 1 0],[0 0 1 1],c1);patch([0 1 1 1-e 1-e 0+e],[0 0 1 1-e 0+e 0+e],c2);patch([0 0 1 1-e 0+e 0+e],[0 1 1 1-e 1-e 0+e],c3);plot([0 1 1 0 0],[0 0 1 1 0]);
  wires:
  "p{5}"/1 -> mux/1
  mux/1 -> "pd{5,4}"/1

== system ball_and_plate_za_nn_2/NARX/Layer 5/LW{5,4} ==
  "ad{5,4}" : Inport  PortDimensions=10  SampleTime=0.001
      mask Display: e = 0.06;c1 = [120 230 180]/255;c2 = ([120 230 180]+0)/(256+128);c3 = ([120 230 180]+128)/(256+128);patch([0 1 1 0],[0 0 1 1],c1);patch([0 1 1 1-e 1-e 0+e],[0 0 1 1-e 0+e 0+e],c2);patch([0 0 1 1-e 0+e 0+e],[0 1 1 1-e 1-e 0+e],c3);plot([0 1 1 0 0],[0 0 1 1 0]);
  "IW{5,4}(1,:)'" : Constant  Value=[-0.5993186560139383001200030776089988648891448974609375;1.15220156548277685715220286510884761810302734375;-1.04801006435799326510505125042982399463653564453125;0.588818598760254108270828510285355150699615478515625;0.81314572435573106989892266938113607466220855712890625;-0.90504484675990093389685853253467939794063568115234375;0.0700781095534457609819156687080976553261280059814453125;0.7012762669828094264090623255469836294651031494140625;-0.207290568772410421782836920101544819772243499755859375;0.62453079569397573767020048762788064777851104736328125]
      mask Display: e = 0.06;c1 = [120 150 230]/255;c2 = ([120 150 230]+0)/383;c3 = ([120 150 230]+128)/383;patch([0 1 1 0],[0 0 1 1],c1);patch([0 1 1 1-e 1-e 0+e],[0 0 1 1-e 0+e 0+e],c2);patch([0 0 1 1-e 0+e 0+e],[0 1 1 1-e 1-e 0+e],c3);plot([0 1 1 0 0],[0 0 1 1 0]);disp('weights');
  Mux : Mux  Inputs=1
      mask Display: e = 0.06;c1 = [120 150 230]/255;c2 = ([120 150 230]+0)/383;c3 = ([120 150 230]+128)/383;patch([0 1 1 0],[0 0 1 1],c1);patch([0 1 1 1-e 1-e 0+e],[0 0 1 1-e 0+e 0+e],c2);patch([0 0 1 1-e 0+e 0+e],[0 1 1 1-e 1-e 0+e],c3);plot([0 1 1 0 0],[0 0 1 1 0]);disp('Mux');
  dotprod1 : neural/Weight Functions/dotprod
  "lz{5,4}" : Outport
      mask Display: e = 0.06;c1 = [120 230 180]/255;c2 = ([120 230 180]+0)/(256+128);c3 = ([120 230 180]+128)/(256+128);patch([0 1 1 0],[0 0 1 1],c1);patch([0 1 1 1-e 1-e 0+e],[0 0 1 1-e 0+e 0+e],c2);patch([0 0 1 1-e 0+e 0+e],[0 1 1 1-e 1-e 0+e],c3);plot([0 1 1 0 0],[0 0 1 1 0]);
  wires:
  "IW{5,4}(1,:)'"/1 -> dotprod1/1
  "ad{5,4}"/1 -> dotprod1/2
  dotprod1/1 -> Mux/1
  Mux/1 -> "lz{5,4}"/1

== system ball_and_plate_za_nn_2/NOE/Layer 1/Delays 1 ==
  "p{1}" : Inport  PortDimensions=1  SampleTime=0.001
      mask Display: e = 0.06;c1 = [120 230 180]/255;c2 = ([120 230 180]+0)/(256+128);c3 = ([120 230 180]+128)/(256+128);patch([0 1 1 0],[0 0 1 1],c1);patch([0 1 1 1-e 1-e 0+e],[0 0 1 1-e 0+e 0+e],c2);patch([0 0 1 1-e 0+e 0+e],[0 1 1 1-e 1-e 0+e],c3);plot([0 1 1 0 0],[0 0 1 1 0]);
  Delay 1 : UnitDelay  InitialCondition=pi_input_1_delayed_1  SampleTime=0.001
      mask Display: e = 0.06;c1 = [120 150 230]/255;c2 = ([120 150 230]+0)/383;c3 = ([120 150 230]+128)/383;patch([0 1 1 0],[0 0 1 1],c1);patch([0 1 1 1-e 1-e 0+e],[0 0 1 1-e 0+e 0+e],c2);patch([0 0 1 1-e 0+e 0+e],[0 1 1 1-e 1-e 0+e],c3);plot([0 1 1 0 0],[0 0 1 1 0]);disp('D')
  Delay 2 : UnitDelay  InitialCondition=pi_input_1_delayed_2  SampleTime=0.001
      mask Display: e = 0.06;c1 = [120 150 230]/255;c2 = ([120 150 230]+0)/383;c3 = ([120 150 230]+128)/383;patch([0 1 1 0],[0 0 1 1],c1);patch([0 1 1 1-e 1-e 0+e],[0 0 1 1-e 0+e 0+e],c2);patch([0 0 1 1-e 0+e 0+e],[0 1 1 1-e 1-e 0+e],c3);plot([0 1 1 0 0],[0 0 1 1 0]);disp('D')
  Delay 3 : UnitDelay  InitialCondition=pi_input_1_delayed_3  SampleTime=0.001
      mask Display: e = 0.06;c1 = [120 150 230]/255;c2 = ([120 150 230]+0)/383;c3 = ([120 150 230]+128)/383;patch([0 1 1 0],[0 0 1 1],c1);patch([0 1 1 1-e 1-e 0+e],[0 0 1 1-e 0+e 0+e],c2);patch([0 0 1 1-e 0+e 0+e],[0 1 1 1-e 1-e 0+e],c3);plot([0 1 1 0 0],[0 0 1 1 0]);disp('D')
  Delay 4 : UnitDelay  InitialCondition=pi_input_1_delayed_4  SampleTime=0.001
      mask Display: e = 0.06;c1 = [120 150 230]/255;c2 = ([120 150 230]+0)/383;c3 = ([120 150 230]+128)/383;patch([0 1 1 0],[0 0 1 1],c1);patch([0 1 1 1-e 1-e 0+e],[0 0 1 1-e 0+e 0+e],c2);patch([0 0 1 1-e 0+e 0+e],[0 1 1 1-e 1-e 0+e],c3);plot([0 1 1 0 0],[0 0 1 1 0]);disp('D')
  Delay 5 : UnitDelay  InitialCondition=pi_input_1_delayed_5  SampleTime=0.001
      mask Display: e = 0.06;c1 = [120 150 230]/255;c2 = ([120 150 230]+0)/383;c3 = ([120 150 230]+128)/383;patch([0 1 1 0],[0 0 1 1],c1);patch([0 1 1 1-e 1-e 0+e],[0 0 1 1-e 0+e 0+e],c2);patch([0 0 1 1-e 0+e 0+e],[0 1 1 1-e 1-e 0+e],c3);plot([0 1 1 0 0],[0 0 1 1 0]);disp('D')
  mux : Mux  Inputs=5
      mask Display: e = 0.06;c1 = [120 150 230]/255;c2 = ([120 150 230]+0)/383;c3 = ([120 150 230]+128)/383;patch([0 1 1 0],[0 0 1 1],c1);patch([0 1 1 1-e 1-e 0+e],[0 0 1 1-e 0+e 0+e],c2);patch([0 0 1 1-e 0+e 0+e],[0 1 1 1-e 1-e 0+e],c3);plot([0 1 1 0 0],[0 0 1 1 0]);disp('Mux')
  "pd{1,1}" : Outport
      mask Display: e = 0.06;c1 = [120 230 180]/255;c2 = ([120 230 180]+0)/(256+128);c3 = ([120 230 180]+128)/(256+128);patch([0 1 1 0],[0 0 1 1],c1);patch([0 1 1 1-e 1-e 0+e],[0 0 1 1-e 0+e 0+e],c2);patch([0 0 1 1-e 0+e 0+e],[0 1 1 1-e 1-e 0+e],c3);plot([0 1 1 0 0],[0 0 1 1 0]);
  wires:
  "p{1}"/1 -> Delay 1/1
  Delay 1/1 -> Delay 2/1, mux/1
  Delay 2/1 -> Delay 3/1, mux/2
  Delay 3/1 -> Delay 4/1, mux/3
  Delay 4/1 -> Delay 5/1, mux/4
  Delay 5/1 -> mux/5
  mux/1 -> "pd{1,1}"/1

== system ball_and_plate_za_nn_2/NOE/Layer 1/Delays 2 ==
  "p{1}" : Inport  PortDimensions=1  SampleTime=0.001
      mask Display: e = 0.06;c1 = [120 230 180]/255;c2 = ([120 230 180]+0)/(256+128);c3 = ([120 230 180]+128)/(256+128);patch([0 1 1 0],[0 0 1 1],c1);patch([0 1 1 1-e 1-e 0+e],[0 0 1 1-e 0+e 0+e],c2);patch([0 0 1 1-e 0+e 0+e],[0 1 1 1-e 1-e 0+e],c3);plot([0 1 1 0 0],[0 0 1 1 0]);
  Delay 1 : UnitDelay  InitialCondition=pi_input_2_delayed_1  SampleTime=0.001
      mask Display: e = 0.06;c1 = [120 150 230]/255;c2 = ([120 150 230]+0)/383;c3 = ([120 150 230]+128)/383;patch([0 1 1 0],[0 0 1 1],c1);patch([0 1 1 1-e 1-e 0+e],[0 0 1 1-e 0+e 0+e],c2);patch([0 0 1 1-e 0+e 0+e],[0 1 1 1-e 1-e 0+e],c3);plot([0 1 1 0 0],[0 0 1 1 0]);disp('D')
  Delay 2 : UnitDelay  InitialCondition=pi_input_2_delayed_2  SampleTime=0.001
      mask Display: e = 0.06;c1 = [120 150 230]/255;c2 = ([120 150 230]+0)/383;c3 = ([120 150 230]+128)/383;patch([0 1 1 0],[0 0 1 1],c1);patch([0 1 1 1-e 1-e 0+e],[0 0 1 1-e 0+e 0+e],c2);patch([0 0 1 1-e 0+e 0+e],[0 1 1 1-e 1-e 0+e],c3);plot([0 1 1 0 0],[0 0 1 1 0]);disp('D')
  Delay 3 : UnitDelay  InitialCondition=pi_input_2_delayed_3  SampleTime=0.001
      mask Display: e = 0.06;c1 = [120 150 230]/255;c2 = ([120 150 230]+0)/383;c3 = ([120 150 230]+128)/383;patch([0 1 1 0],[0 0 1 1],c1);patch([0 1 1 1-e 1-e 0+e],[0 0 1 1-e 0+e 0+e],c2);patch([0 0 1 1-e 0+e 0+e],[0 1 1 1-e 1-e 0+e],c3);plot([0 1 1 0 0],[0 0 1 1 0]);disp('D')
  Delay 4 : UnitDelay  InitialCondition=pi_input_2_delayed_4  SampleTime=0.001
      mask Display: e = 0.06;c1 = [120 150 230]/255;c2 = ([120 150 230]+0)/383;c3 = ([120 150 230]+128)/383;patch([0 1 1 0],[0 0 1 1],c1);patch([0 1 1 1-e 1-e 0+e],[0 0 1 1-e 0+e 0+e],c2);patch([0 0 1 1-e 0+e 0+e],[0 1 1 1-e 1-e 0+e],c3);plot([0 1 1 0 0],[0 0 1 1 0]);disp('D')
  Delay 5 : UnitDelay  InitialCondition=pi_input_2_delayed_5  SampleTime=0.001
      mask Display: e = 0.06;c1 = [120 150 230]/255;c2 = ([120 150 230]+0)/383;c3 = ([120 150 230]+128)/383;patch([0 1 1 0],[0 0 1 1],c1);patch([0 1 1 1-e 1-e 0+e],[0 0 1 1-e 0+e 0+e],c2);patch([0 0 1 1-e 0+e 0+e],[0 1 1 1-e 1-e 0+e],c3);plot([0 1 1 0 0],[0 0 1 1 0]);disp('D')
  mux : Mux  Inputs=5
      mask Display: e = 0.06;c1 = [120 150 230]/255;c2 = ([120 150 230]+0)/383;c3 = ([120 150 230]+128)/383;patch([0 1 1 0],[0 0 1 1],c1);patch([0 1 1 1-e 1-e 0+e],[0 0 1 1-e 0+e 0+e],c2);patch([0 0 1 1-e 0+e 0+e],[0 1 1 1-e 1-e 0+e],c3);plot([0 1 1 0 0],[0 0 1 1 0]);disp('Mux')
  "pd{1,2}" : Outport
      mask Display: e = 0.06;c1 = [120 230 180]/255;c2 = ([120 230 180]+0)/(256+128);c3 = ([120 230 180]+128)/(256+128);patch([0 1 1 0],[0 0 1 1],c1);patch([0 1 1 1-e 1-e 0+e],[0 0 1 1-e 0+e 0+e],c2);patch([0 0 1 1-e 0+e 0+e],[0 1 1 1-e 1-e 0+e],c3);plot([0 1 1 0 0],[0 0 1 1 0]);
  wires:
  "p{1}"/1 -> Delay 1/1
  Delay 1/1 -> Delay 2/1, mux/1
  Delay 2/1 -> Delay 3/1, mux/2
  Delay 3/1 -> Delay 4/1, mux/3
  Delay 4/1 -> Delay 5/1, mux/4
  Delay 5/1 -> mux/5
  mux/1 -> "pd{1,2}"/1
